simulink model "MOT_CTRL_PWM_FUN_001"  (R2025a)
settings: Solver=FixedStepAuto  StartTime=0.0  StopTime=10  FixedStep=1e-4  RelTol=1e-3
libraries: simulink x2
settings Model: DataDictionary=PwmGenerator.sldd  Creator=tecnicomcbti  LastModifiedBy=tecnicomcbti

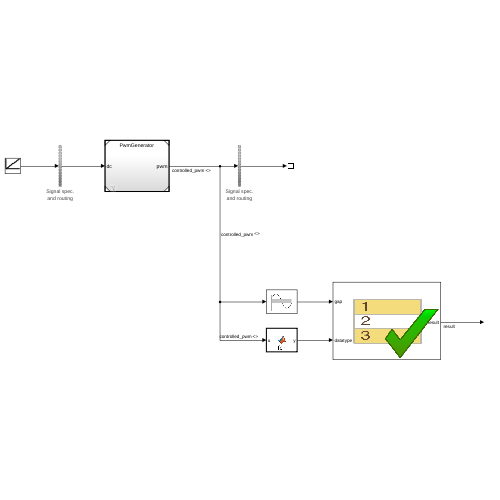
[thumbnail: Simulink's stored preview of the top-level diagram]
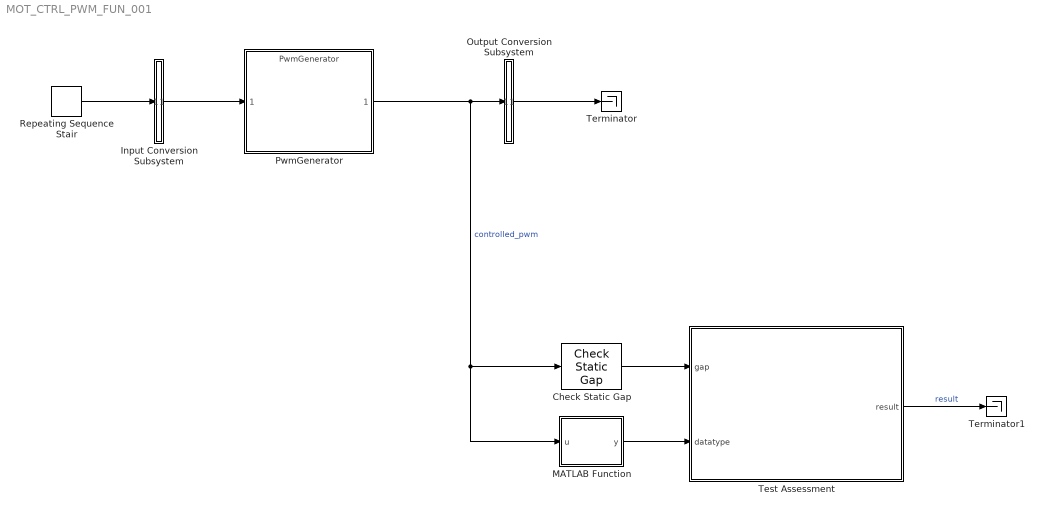
== system MOT_CTRL_PWM_FUN_001 ==
  Check Static Gap : simulink/Model Verification/Check  Static Gap  Description=u <= 0 || 5 <= u  max=5  max_included=on  min=0  min_included=on  enabled=on  stopWhenAssertionFail=off  export=on  icon=graphic
  Input Conversion Subsystem : Subsystem  Tag=__SLT_ICS__  Description=|
      | Signal spec.
      | and routing
      settings: AttributesFormatString=%<Description>
  MATLAB Function : MATLAB Function  TreatAsAtomicUnit=on
  Output Conversion Subsystem : Subsystem  Tag=__SLT_OCS__  Description=|
      | Signal spec.
      | and routing
      settings: AttributesFormatString=%<Description>
  PwmGenerator : ModelReference  ModelNameDialog=PwmGenerator  SimulationMode=Normal  ModelReferenceVersion=1.9
  Repeating Sequence Stair : simulink/Sources/Repeating Sequence Stair  OutValues=(1/100).*[0, 10, 20, 30, 40, 50, 60, 70, 80, 90, 100].'  tsamp=1/2  OutMin=[]  OutMax=[]  OutDataTypeStr=double  OutputDataTypeScalingMode=double  OutDataType=fixdt(0,8)  ConRadixGroup=Best Precision: Vector-wise  OutScaling=2^-12
  Terminator : Terminator
  Terminator1 : Terminator
  Test Assessment : Test Sequence  TreatAsAtomicUnit=on
  wires:
  Input Conversion Subsystem/1(Outport_1) -> PwmGenerator/1
  Output Conversion Subsystem/1(Outport_1) -> Terminator/1
  MATLAB Function/1(y) -> Test Assessment/2(datatype)
  Test Assessment/1(result) -> Terminator1/1  "result"
  PwmGenerator/1 -> Check Static Gap/1, MATLAB Function/1(u), Output Conversion Subsystem/1(Inport_1)  "controlled_pwm"
  Check Static Gap/1 -> Test Assessment/1(gap)
  Repeating Sequence Stair/1 -> Input Conversion Subsystem/1(Inport_1)

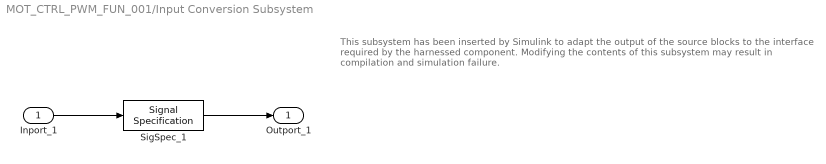
== system MOT_CTRL_PWM_FUN_001/Input Conversion Subsystem ==
  note: This subsystem has been inserted by Simulink to adapt the output of the source blocks to the interface required by the harnessed component.
      |  Modifying the contents of this subsystem may result in compilation and simulation failure.
  Inport_1 : Inport
  SigSpec_1 : SignalSpecification  OutDataTypeStr=double  Dimensions=[1]  SampleTime=0.0001
  Outport_1 : Outport
  wires:
  SigSpec_1/1 -> Outport_1/1
  Inport_1/1 -> SigSpec_1/1

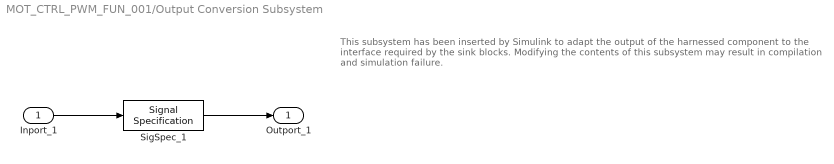
== system MOT_CTRL_PWM_FUN_001/Output Conversion Subsystem ==
  note: This subsystem has been inserted by Simulink to adapt the output of the harnessed component to the interface required by the sink blocks.
      |  Modifying the contents of this subsystem may result in compilation and simulation failure.
  Inport_1 : Inport
  SigSpec_1 : SignalSpecification  OutDataTypeStr=double  Dimensions=[1]  SampleTime=0.0001
  Outport_1 : Outport
  wires:
  Inport_1/1 -> SigSpec_1/1
  SigSpec_1/1 -> Outport_1/1

== stateflow chart MOT_CTRL_PWM_FUN_001/Test Assessment ==
  state Init
    state CheckGapAndType
      result = true;
    state else
      result = false;
    (default) -> (junction 22)
    Init -> (junction 22)
    (junction 22) -> (junction 23) [order 1] : [(gap == true && datatype == 1)
        | ]
    (junction 23) -> CheckGapAndType [order 1] : [~in(Init.CheckGapAndType)]
    (junction 23) -> (junction 26) [order 2]
    (junction 31) -> (junction 32)
    (junction 32) -> else [order 1] : [~in(Init.else)]
    (junction 32) -> (junction 35) [order 2]
    (junction 22) -> (junction 31) [order 2]
  (default) -> Init
  data: gap input boolean size=1; datatype input uint8 size=1; result output boolean size=1

== matlab function MOT_CTRL_PWM_FUN_001/MATLAB Function ==
  data: u input; y output
function y = fcn(u)
    data_type = class(u);
    
    switch data_type
        case 'double'
            y = uint8(1);
        case 'single'
            y = uint8(2);
        case 'int8'
            y = uint8(3);
        case 'uint8'
            y = uint8(4);
        case 'int16'
            y = uint8(5);
        case 'uint16'
            y = uint8(6);
        case 'int32'
            y = uint8(7);
        case 'uint32'
            y = uint8(8);
        case 'int64'
            y = uint8(9);
        case 'uint64'
            y = uint8(10);
        case 'logical'
            y = uint8(11);
        otherwise
            y = uint8(0); % Tipo desconhecido
    end
end
